simulink model "testProject2"  (R2017a)
settings: Solver=VariableStepAuto  StartTime=0.0  StopTime=inf  RelTol=1e-3
libraries: libraryProject2 x4, realtime_pacer_lib x1
settings Model: Creator=ibrahim  LastModifiedBy=ibrahim

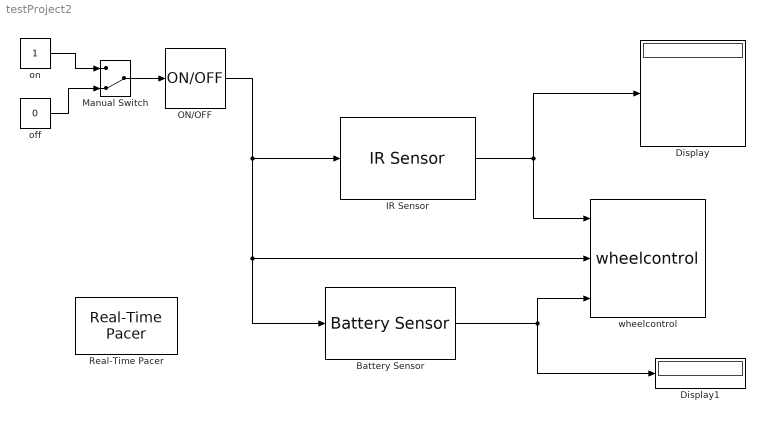
== system testProject2 ==
  Battery Sensor : libraryProject2/Battery Sensor
  Display : Display
  Display1 : Display
  IR Sensor : libraryProject2/IR Sensor
  Manual Switch : ManualSwitch  CurrentSetting=0
  ON/OFF : libraryProject2/ON//OFF
  Real-Time Pacer : realtime_pacer_lib/Real-Time Pacer  simTimePerRealTime=.5
  off : Constant  Value=0
  on : Constant
  wheelcontrol : libraryProject2/wheelcontrol
  wires:
  ON/OFF/1 -> IR Sensor/1, wheelcontrol/2, Battery Sensor/1
  IR Sensor/1 -> wheelcontrol/1, Display/1
  Battery Sensor/1 -> Display1/1, wheelcontrol/3
  Manual Switch/1 -> ON/OFF/1
  on/1 -> Manual Switch/1
  off/1 -> Manual Switch/2
